simulink model "SM_Offshore_Windturbine"  (R2021a)
settings: Solver=ode4  StartTime=0.0  StopTime=par.sym.Ttot  FixedStep=par.sym.max_dt  MaxStep=par.sym.max_dt  RelTol=1e-3
model workspace: external: MATLAB File C:\Users\d053704\Desktop\MOST\Structure\CAD\CAD_DataFile.m (data not in the file)
undefined symbols (not defined in the file): par, smiData, X, Y, Z
libraries: sm_lib x50, simulink_extras x29, vrlib x18, nesl_utility x10, dspstat3 x9, sharedutil x5, eeGeneralControl x2
(part 4 of 4)

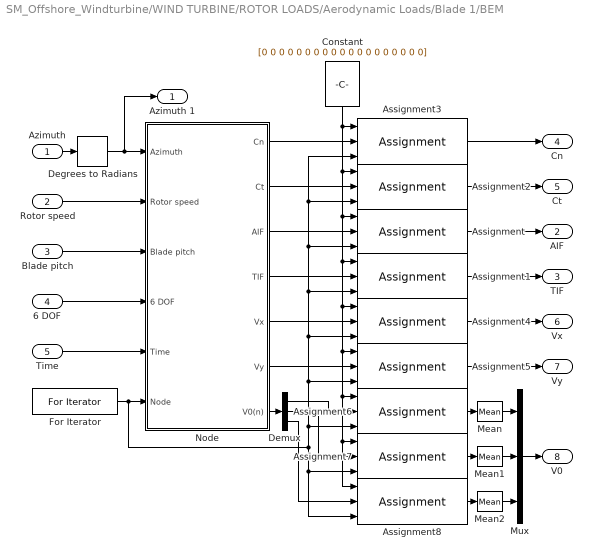
== system SM_Offshore_Windturbine/WIND TURBINE/ROTOR LOADS/Aerodynamic Loads/Blade 1/BEM ==
  Azimuth : Inport
  Rotor speed : Inport  Port=2
  Blade pitch : Inport  Port=3
  6 DOF : Inport  Port=4
  Time : Inport  Port=5
  Assignment{,1..8} (9 alike) : Assignment  IndexOptions=Index vector (port)  Indices=1  OutputSizes=1
  Constant : Constant  Value=[0 0 0 0 0 0 0 0 0 0 0 0 0 0 0 0 0 0 0]
  Degrees to Radians : simulink_extras/Transformations/Degrees to Radians
  Demux : Demux  Outputs=3
  For Iterator : ForIterator  IterationLimit=19  IterationVariableDataType=double
  Mean : dspstat3/Mean  run=off  InputProcessing=Columns as channels (frame based)  reset_popup=None  directionMode=Each column  dimension=1  roiEnable=off  roiType=Rectangles  roiPortion=Entire ROI  roiOutput=Individual statistics for each ROI  roiFlag=off  roundingMode=Floor  overflowMode=off  outputDataTypeStr=Inherit: Same as accumulator  outputMin=[]  outputMax=[]  outputLastDataTypeStr=Inherit: Same as accumulator
  Mean1 : dspstat3/Mean  run=off  InputProcessing=Columns as channels (frame based)  reset_popup=None  directionMode=Each column  dimension=1  roiEnable=off  roiType=Rectangles  roiPortion=Entire ROI  roiOutput=Individual statistics for each ROI  roiFlag=off  roundingMode=Floor  overflowMode=off  outputDataTypeStr=Inherit: Same as accumulator  outputMin=[]  outputMax=[]  outputLastDataTypeStr=Inherit: Same as accumulator
  Mean2 : dspstat3/Mean  run=off  InputProcessing=Columns as channels (frame based)  reset_popup=None  directionMode=Each column  dimension=1  roiEnable=off  roiType=Rectangles  roiPortion=Entire ROI  roiOutput=Individual statistics for each ROI  roiFlag=off  roundingMode=Floor  overflowMode=off  outputDataTypeStr=Inherit: Same as accumulator  outputMin=[]  outputMax=[]  outputLastDataTypeStr=Inherit: Same as accumulator
  Mux : Mux  Inputs=3
  Node : Subsystem
  Azimuth 1 : Outport  VectorParamsAs1DForOutWhenUnconnected=off
  AIF : Outport  Port=2  VectorParamsAs1DForOutWhenUnconnected=off
  TIF : Outport  Port=3  VectorParamsAs1DForOutWhenUnconnected=off
  Cn : Outport  Port=4  VectorParamsAs1DForOutWhenUnconnected=off
  Ct : Outport  Port=5  VectorParamsAs1DForOutWhenUnconnected=off
  Vx : Outport  Port=6  VectorParamsAs1DForOutWhenUnconnected=off
  Vy : Outport  Port=7  VectorParamsAs1DForOutWhenUnconnected=off
  V0 : Outport  Port=8  VectorParamsAs1DForOutWhenUnconnected=off
  wires:
  Blade pitch/1 -> Node/3(Blade pitch)
  6 DOF/1 -> Node/4(6 DOF)
  Time/1 -> Node/5(Time)
  Rotor speed/1 -> Node/2(Rotor speed)
  For Iterator/1 -> Node/6(Node), Assignment8/3, Assignment7/3, Assignment6/3, Assignment5/3, Assignment1/3, Assignment/3, Assignment3/3, Assignment2/3, Assignment4/3
  Assignment/1 -> AIF/1
  Assignment1/1 -> TIF/1
  Node/3(AIF) -> Assignment/2
  Node/4(TIF) -> Assignment1/2
  Node/2(Ct) -> Assignment2/2
  Node/1(Cn) -> Assignment3/2
  Node/5(Vx) -> Assignment4/2
  Node/6(Vy) -> Assignment5/2
  Constant/1 -> Assignment7/1, Assignment8/1, Assignment6/1, Assignment5/1, Assignment4/1, Assignment1/1, Assignment/1, Assignment2/1, Assignment3/1
  Assignment3/1 -> Cn/1
  Assignment2/1 -> Ct/1
  Assignment4/1 -> Vx/1
  Assignment5/1 -> Vy/1
  Node/7(V0(n)) -> Demux/1
  Demux/1 -> Assignment6/2
  Demux/3 -> Assignment8/2
  Demux/2 -> Assignment7/2
  Mux/1 -> V0/1
  Assignment6/1 -> Mean/1
  Assignment7/1 -> Mean1/1
  Assignment8/1 -> Mean2/1
  Mean/1 -> Mux/1
  Mean1/1 -> Mux/2
  Mean2/1 -> Mux/3
  Azimuth/1 -> Degrees to Radians/1
  Degrees to Radians/1 -> Node/1(Azimuth), Azimuth 1/1

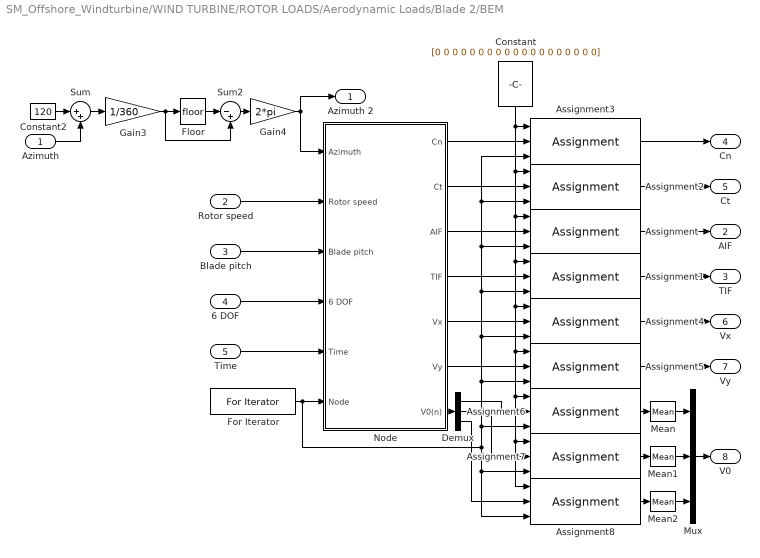
== system SM_Offshore_Windturbine/WIND TURBINE/ROTOR LOADS/Aerodynamic Loads/Blade 2/BEM ==
  Azimuth : Inport
  Rotor speed : Inport  Port=2
  Blade pitch : Inport  Port=3
  6 DOF : Inport  Port=4
  Time : Inport  Port=5
  Assignment{,1..8} (9 alike) : Assignment  IndexOptions=Index vector (port)  Indices=1  OutputSizes=1
  Constant : Constant  Value=[0 0 0 0 0 0 0 0 0 0 0 0 0 0 0 0 0 0 0]
  Constant2 : Constant  Value=120
  Demux : Demux  Outputs=3
  Floor : Rounding
  For Iterator : ForIterator  IterationLimit=19  IterationVariableDataType=double
  Gain3 : Gain  Gain=1/360
  Gain4 : Gain  Gain=2*pi
  Mean : dspstat3/Mean  run=off  InputProcessing=Columns as channels (frame based)  reset_popup=None  directionMode=Each column  dimension=1  roiEnable=off  roiType=Rectangles  roiPortion=Entire ROI  roiOutput=Individual statistics for each ROI  roiFlag=off  roundingMode=Floor  overflowMode=off  outputDataTypeStr=Inherit: Same as accumulator  outputMin=[]  outputMax=[]  outputLastDataTypeStr=Inherit: Same as accumulator
  Mean1 : dspstat3/Mean  run=off  InputProcessing=Columns as channels (frame based)  reset_popup=None  directionMode=Each column  dimension=1  roiEnable=off  roiType=Rectangles  roiPortion=Entire ROI  roiOutput=Individual statistics for each ROI  roiFlag=off  roundingMode=Floor  overflowMode=off  outputDataTypeStr=Inherit: Same as accumulator  outputMin=[]  outputMax=[]  outputLastDataTypeStr=Inherit: Same as accumulator
  Mean2 : dspstat3/Mean  run=off  InputProcessing=Columns as channels (frame based)  reset_popup=None  directionMode=Each column  dimension=1  roiEnable=off  roiType=Rectangles  roiPortion=Entire ROI  roiOutput=Individual statistics for each ROI  roiFlag=off  roundingMode=Floor  overflowMode=off  outputDataTypeStr=Inherit: Same as accumulator  outputMin=[]  outputMax=[]  outputLastDataTypeStr=Inherit: Same as accumulator
  Mux : Mux  Inputs=3
  Node : Subsystem
  Sum : Sum  Inputs=|++
  Sum2 : Sum  Inputs=|-+
  Azimuth 2 : Outport  VectorParamsAs1DForOutWhenUnconnected=off
  AIF : Outport  Port=2  VectorParamsAs1DForOutWhenUnconnected=off
  TIF : Outport  Port=3  VectorParamsAs1DForOutWhenUnconnected=off
  Cn : Outport  Port=4  VectorParamsAs1DForOutWhenUnconnected=off
  Ct : Outport  Port=5  VectorParamsAs1DForOutWhenUnconnected=off
  Vx : Outport  Port=6  VectorParamsAs1DForOutWhenUnconnected=off
  Vy : Outport  Port=7  VectorParamsAs1DForOutWhenUnconnected=off
  V0 : Outport  Port=8  VectorParamsAs1DForOutWhenUnconnected=off
  wires:
  Blade pitch/1 -> Node/3(Blade pitch)
  6 DOF/1 -> Node/4(6 DOF)
  Time/1 -> Node/5(Time)
  Rotor speed/1 -> Node/2(Rotor speed)
  Sum/1 -> Gain3/1
  Floor/1 -> Sum2/1
  Constant2/1 -> Sum/1
  Gain3/1 -> Sum2/2, Floor/1
  Sum2/1 -> Gain4/1
  Gain4/1 -> Node/1(Azimuth), Azimuth 2/1
  Azimuth/1 -> Sum/2
  Mean/1 -> Mux/1
  Node/7(V0(n)) -> Demux/1
  Node/5(Vx) -> Assignment4/2
  Mux/1 -> V0/1
  Assignment5/1 -> Vy/1
  Assignment4/1 -> Vx/1
  Constant/1 -> Assignment7/1, Assignment8/1, Assignment6/1, Assignment5/1, Assignment4/1, Assignment1/1, Assignment/1, Assignment2/1, Assignment3/1
  Demux/2 -> Assignment7/2
  Mean2/1 -> Mux/3
  Assignment8/1 -> Mean2/1
  Assignment6/1 -> Mean/1
  Assignment/1 -> AIF/1
  Node/4(TIF) -> Assignment1/2
  Assignment1/1 -> TIF/1
  Node/3(AIF) -> Assignment/2
  Demux/1 -> Assignment6/2
  Demux/3 -> Assignment8/2
  For Iterator/1 -> Node/6(Node), Assignment8/3, Assignment7/3, Assignment6/3, Assignment5/3, Assignment1/3, Assignment/3, Assignment3/3, Assignment2/3, Assignment4/3
  Node/2(Ct) -> Assignment2/2
  Node/1(Cn) -> Assignment3/2
  Assignment2/1 -> Ct/1
  Assignment3/1 -> Cn/1
  Node/6(Vy) -> Assignment5/2
  Mean1/1 -> Mux/2
  Assignment7/1 -> Mean1/1

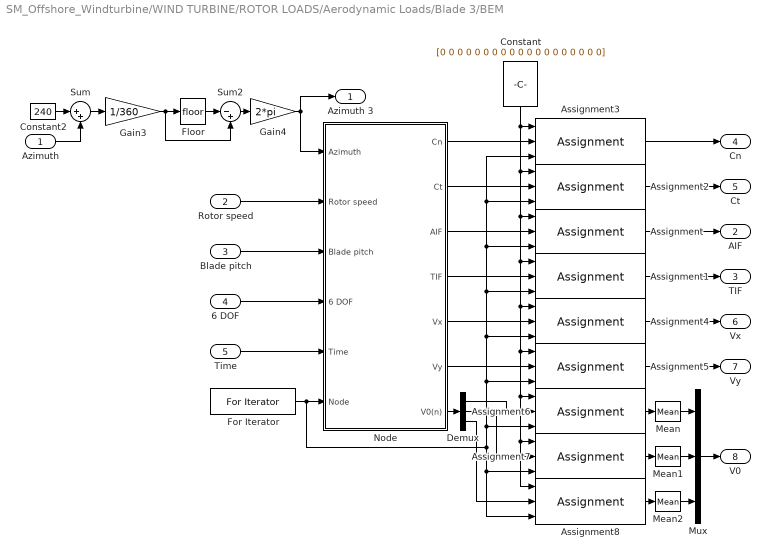
== system SM_Offshore_Windturbine/WIND TURBINE/ROTOR LOADS/Aerodynamic Loads/Blade 3/BEM ==
  Azimuth : Inport
  Rotor speed : Inport  Port=2
  Blade pitch : Inport  Port=3
  6 DOF : Inport  Port=4
  Time : Inport  Port=5
  Assignment{,1..8} (9 alike) : Assignment  IndexOptions=Index vector (port)  Indices=1  OutputSizes=1
  Constant : Constant  Value=[0 0 0 0 0 0 0 0 0 0 0 0 0 0 0 0 0 0 0]
  Constant2 : Constant  Value=240
  Demux : Demux  Outputs=3
  Floor : Rounding
  For Iterator : ForIterator  IterationLimit=19  IterationVariableDataType=double
  Gain3 : Gain  Gain=1/360
  Gain4 : Gain  Gain=2*pi
  Mean : dspstat3/Mean  run=off  InputProcessing=Columns as channels (frame based)  reset_popup=None  directionMode=Each column  dimension=1  roiEnable=off  roiType=Rectangles  roiPortion=Entire ROI  roiOutput=Individual statistics for each ROI  roiFlag=off  roundingMode=Floor  overflowMode=off  outputDataTypeStr=Inherit: Same as accumulator  outputMin=[]  outputMax=[]  outputLastDataTypeStr=Inherit: Same as accumulator
  Mean1 : dspstat3/Mean  run=off  InputProcessing=Columns as channels (frame based)  reset_popup=None  directionMode=Each column  dimension=1  roiEnable=off  roiType=Rectangles  roiPortion=Entire ROI  roiOutput=Individual statistics for each ROI  roiFlag=off  roundingMode=Floor  overflowMode=off  outputDataTypeStr=Inherit: Same as accumulator  outputMin=[]  outputMax=[]  outputLastDataTypeStr=Inherit: Same as accumulator
  Mean2 : dspstat3/Mean  run=off  InputProcessing=Columns as channels (frame based)  reset_popup=None  directionMode=Each column  dimension=1  roiEnable=off  roiType=Rectangles  roiPortion=Entire ROI  roiOutput=Individual statistics for each ROI  roiFlag=off  roundingMode=Floor  overflowMode=off  outputDataTypeStr=Inherit: Same as accumulator  outputMin=[]  outputMax=[]  outputLastDataTypeStr=Inherit: Same as accumulator
  Mux : Mux  Inputs=3
  Node : Subsystem
  Sum : Sum  Inputs=|++
  Sum2 : Sum  Inputs=|-+
  Azimuth 3 : Outport  VectorParamsAs1DForOutWhenUnconnected=off
  AIF : Outport  Port=2  VectorParamsAs1DForOutWhenUnconnected=off
  TIF : Outport  Port=3  VectorParamsAs1DForOutWhenUnconnected=off
  Cn : Outport  Port=4  VectorParamsAs1DForOutWhenUnconnected=off
  Ct : Outport  Port=5  VectorParamsAs1DForOutWhenUnconnected=off
  Vx : Outport  Port=6  VectorParamsAs1DForOutWhenUnconnected=off
  Vy : Outport  Port=7  VectorParamsAs1DForOutWhenUnconnected=off
  V0 : Outport  Port=8  VectorParamsAs1DForOutWhenUnconnected=off
  wires:
  Azimuth/1 -> Sum/2
  Gain4/1 -> Node/1(Azimuth), Azimuth 3/1
  Sum2/1 -> Gain4/1
  Gain3/1 -> Floor/1, Sum2/2
  Constant2/1 -> Sum/1
  Floor/1 -> Sum2/1
  Sum/1 -> Gain3/1
  Rotor speed/1 -> Node/2(Rotor speed)
  Time/1 -> Node/5(Time)
  6 DOF/1 -> Node/4(6 DOF)
  Blade pitch/1 -> Node/3(Blade pitch)
  Mean/1 -> Mux/1
  Node/7(V0(n)) -> Demux/1
  Node/5(Vx) -> Assignment4/2
  Mux/1 -> V0/1
  Assignment5/1 -> Vy/1
  Assignment4/1 -> Vx/1
  Constant/1 -> Assignment7/1, Assignment8/1, Assignment6/1, Assignment5/1, Assignment4/1, Assignment1/1, Assignment/1, Assignment2/1, Assignment3/1
  Demux/2 -> Assignment7/2
  Mean2/1 -> Mux/3
  Assignment8/1 -> Mean2/1
  Assignment6/1 -> Mean/1
  Assignment/1 -> AIF/1
  Node/4(TIF) -> Assignment1/2
  Assignment1/1 -> TIF/1
  Node/3(AIF) -> Assignment/2
  Demux/1 -> Assignment6/2
  Demux/3 -> Assignment8/2
  For Iterator/1 -> Node/6(Node), Assignment8/3, Assignment7/3, Assignment6/3, Assignment5/3, Assignment1/3, Assignment/3, Assignment3/3, Assignment2/3, Assignment4/3
  Node/2(Ct) -> Assignment2/2
  Node/1(Cn) -> Assignment3/2
  Assignment2/1 -> Ct/1
  Assignment3/1 -> Cn/1
  Node/6(Vy) -> Assignment5/2
  Mean1/1 -> Mux/2
  Assignment7/1 -> Mean1/1

== system SM_Offshore_Windturbine/WIND TURBINE/ROTOR LOADS/TowerBaseLoads/3D rotation matrix/If Action Subsystem ==
  Action Port : ActionPort  ActionPortLabel=if(u1 == 0)
  Constant : Constant  Value=[1 0 0; 0 1 0; 0 0 1]
  R : Outport  VectorParamsAs1DForOutWhenUnconnected=off
  wires:
  Constant/1 -> R/1

== system SM_Offshore_Windturbine/WIND TURBINE/ROTOR LOADS/TowerBaseLoads/3D rotation matrix/If Action Subsystem1 ==
  TETA : Inport
  rad : Inport  Port=2
  T : Inport  Port=3
  Action Port : ActionPort  ActionPortLabel=else
  Divide : Product  Inputs=//*
  R : Outport  VectorParamsAs1DForOutWhenUnconnected=off
  wires:
  T/1 -> Divide/3
  TETA/1 -> Divide/1
  rad/1 -> Divide/2
  Divide/1 -> R/1

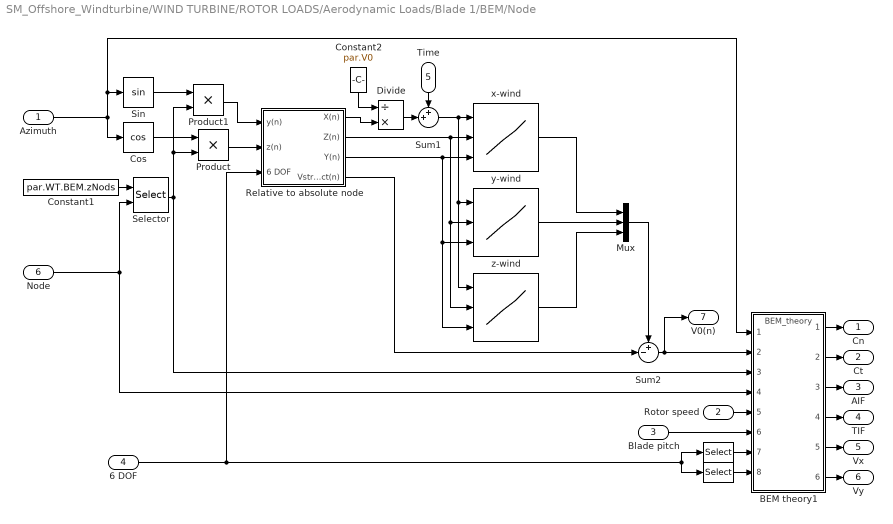
== system SM_Offshore_Windturbine/WIND TURBINE/ROTOR LOADS/Aerodynamic Loads/Blade 1/BEM/Node ==
  Azimuth : Inport
  Rotor speed : Inport  Port=2
  Blade pitch : Inport  Port=3
  6 DOF : Inport  Port=4
  Time : Inport  Port=5
  Node : Inport  Port=6
  " " : Selector  InputPortWidth=18  IndexOptions=Index vector (dialog)  Indices=6  OutputSizes=1
  "  " : Selector  InputPortWidth=18  IndexOptions=Index vector (dialog)  Indices=5  OutputSizes=1
  BEM theory1 : ModelReference  ModelNameDialog=BEM_theory.slxp  ModelReferenceVersion=5.17  CopyOfModelProtected=on
  Constant1 : Constant  Value=par.WT.BEM.zNods
  Constant2 : Constant  Value=par.V0  VectorParams1D=off
  Cos : Trigonometry  Operator=cos
  Divide : Product  Inputs=/*
  Mux : Mux  Inputs=3
  Product : Product
  Product1 : Product
  Relative to absolute node : Subsystem
  Selector : Selector  InputPortWidth=19  IndexOptions=Index vector (port)  Indices=Node  OutputSizes=1
  Sin : Trigonometry
  Sum1 : Sum  Inputs=++|
  Sum2 : Sum  Inputs=+-|
  x-wind : Lookup_n-D  NumberOfTableDimensions=3  BreakpointsForDimension1=par.wind.Time  BreakpointsForDimension2=par.wind.Zdiscr  BreakpointsForDimension3=par.wind.Ydiscr  BreakpointsForDimension4=par.WT.BEM.WINDANGLE  BreakpointsForDimension5=par.WT.BEM.AZIMUTH  BreakpointsForDimension6=par.WT.BEM.YAW  Table=par.wind.SpatialDiscrU  DiagnosticForOutOfRangeInput=Warning  RndMeth=Simplest  InputSameDT=on
      settings: InputPortMap=u0,u1,u2
  y-wind : Lookup_n-D  NumberOfTableDimensions=3  BreakpointsForDimension1=par.wind.Time  BreakpointsForDimension2=par.wind.Zdiscr  BreakpointsForDimension3=par.wind.Ydiscr  BreakpointsForDimension4=par.WT.BEM.WINDANGLE  BreakpointsForDimension5=par.WT.BEM.AZIMUTH  BreakpointsForDimension6=par.WT.BEM.YAW  Table=par.wind.SpatialDiscrV  DiagnosticForOutOfRangeInput=Warning  RndMeth=Simplest  InputSameDT=on
      settings: InputPortMap=u0,u1,u2
  z-wind : Lookup_n-D  NumberOfTableDimensions=3  BreakpointsForDimension1=par.wind.Time  BreakpointsForDimension2=par.wind.Zdiscr  BreakpointsForDimension3=par.wind.Ydiscr  BreakpointsForDimension4=par.WT.BEM.WINDANGLE  BreakpointsForDimension5=par.WT.BEM.AZIMUTH  BreakpointsForDimension6=par.WT.BEM.YAW  Table=par.wind.SpatialDiscrW  DiagnosticForOutOfRangeInput=Warning  RndMeth=Simplest  InputSameDT=on
      settings: InputPortMap=u0,u1,u2
  Cn : Outport  VectorParamsAs1DForOutWhenUnconnected=off
  Ct : Outport  Port=2  VectorParamsAs1DForOutWhenUnconnected=off
  AIF : Outport  Port=3  VectorParamsAs1DForOutWhenUnconnected=off
  TIF : Outport  Port=4  VectorParamsAs1DForOutWhenUnconnected=off
  Vx : Outport  Port=5  VectorParamsAs1DForOutWhenUnconnected=off
  Vy : Outport  Port=6  VectorParamsAs1DForOutWhenUnconnected=off
  V0(n) : Outport  Port=7  VectorParamsAs1DForOutWhenUnconnected=off
  wires:
  BEM theory1/2 -> Ct/1
  BEM theory1/1 -> Cn/1
  Divide/1 -> Sum1/2
  Product/1 -> Relative to absolute node/2(z(n))
  Cos/1 -> Product/1
  x-wind/1 -> Mux/1
  Product1/1 -> Relative to absolute node/1(y(n))
  y-wind/1 -> Mux/2
  Relative to absolute node/1(X(n)) -> Divide/2
  Relative to absolute node/3(Y(n)) -> x-wind/3, z-wind/3, y-wind/3
  Sum1/1 -> z-wind/1, y-wind/1, x-wind/1
  Constant2/1 -> Divide/1
  Azimuth/1 -> BEM theory1/1, Sin/1, Cos/1
  Selector/1 -> BEM theory1/3, Product/2, Product1/2
  z-wind/1 -> Mux/3
  Sin/1 -> Product1/1
  "  "/1 -> BEM theory1/7
  " "/1 -> BEM theory1/8
  Rotor speed/1 -> BEM theory1/5
  6 DOF/1 -> Relative to absolute node/3(6 DOF), " "/1, "  "/1
  Blade pitch/1 -> BEM theory1/6
  Node/1 -> BEM theory1/4, Selector/2
  Constant1/1 -> Selector/1
  Time/1 -> Sum1/1
  BEM theory1/3 -> AIF/1
  Relative to absolute node/4(Vstruct(n)) -> Sum2/2
  BEM theory1/4 -> TIF/1
  BEM theory1/6 -> Vy/1
  BEM theory1/5 -> Vx/1
  Sum2/1 -> BEM theory1/2, V0(n)/1
  Relative to absolute node/2(Z(n)) -> z-wind/2, y-wind/2, x-wind/2
  Mux/1 -> Sum2/1

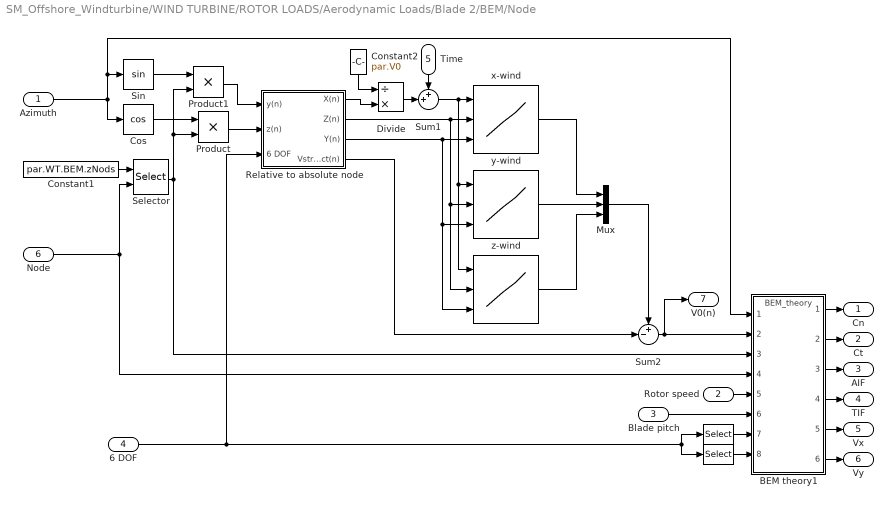
== system SM_Offshore_Windturbine/WIND TURBINE/ROTOR LOADS/Aerodynamic Loads/Blade 2/BEM/Node ==
  Azimuth : Inport
  Rotor speed : Inport  Port=2
  Blade pitch : Inport  Port=3
  6 DOF : Inport  Port=4
  Time : Inport  Port=5
  Node : Inport  Port=6
  " " : Selector  InputPortWidth=18  IndexOptions=Index vector (dialog)  Indices=6  OutputSizes=1
  "  " : Selector  InputPortWidth=18  IndexOptions=Index vector (dialog)  Indices=5  OutputSizes=1
  BEM theory1 : ModelReference  ModelNameDialog=BEM_theory.slxp  ModelReferenceVersion=5.17  CopyOfModelProtected=on
  Constant1 : Constant  Value=par.WT.BEM.zNods
  Constant2 : Constant  Value=par.V0  VectorParams1D=off
  Cos : Trigonometry  Operator=cos
  Divide : Product  Inputs=/*
  Mux : Mux  Inputs=3
  Product : Product
  Product1 : Product
  Relative to absolute node : Subsystem
  Selector : Selector  InputPortWidth=19  IndexOptions=Index vector (port)  Indices=Node  OutputSizes=1
  Sin : Trigonometry
  Sum1 : Sum  Inputs=++|
  Sum2 : Sum  Inputs=+-|
  x-wind : Lookup_n-D  NumberOfTableDimensions=3  BreakpointsForDimension1=par.wind.Time  BreakpointsForDimension2=par.wind.Zdiscr  BreakpointsForDimension3=par.wind.Ydiscr  BreakpointsForDimension4=par.WT.BEM.WINDANGLE  BreakpointsForDimension5=par.WT.BEM.AZIMUTH  BreakpointsForDimension6=par.WT.BEM.YAW  Table=par.wind.SpatialDiscrU  DiagnosticForOutOfRangeInput=Warning  RndMeth=Simplest  InputSameDT=on
      settings: InputPortMap=u0,u1,u2
  y-wind : Lookup_n-D  NumberOfTableDimensions=3  BreakpointsForDimension1=par.wind.Time  BreakpointsForDimension2=par.wind.Zdiscr  BreakpointsForDimension3=par.wind.Ydiscr  BreakpointsForDimension4=par.WT.BEM.WINDANGLE  BreakpointsForDimension5=par.WT.BEM.AZIMUTH  BreakpointsForDimension6=par.WT.BEM.YAW  Table=par.wind.SpatialDiscrV  DiagnosticForOutOfRangeInput=Warning  RndMeth=Simplest  InputSameDT=on
      settings: InputPortMap=u0,u1,u2
  z-wind : Lookup_n-D  NumberOfTableDimensions=3  BreakpointsForDimension1=par.wind.Time  BreakpointsForDimension2=par.wind.Zdiscr  BreakpointsForDimension3=par.wind.Ydiscr  BreakpointsForDimension4=par.WT.BEM.WINDANGLE  BreakpointsForDimension5=par.WT.BEM.AZIMUTH  BreakpointsForDimension6=par.WT.BEM.YAW  Table=par.wind.SpatialDiscrW  DiagnosticForOutOfRangeInput=Warning  RndMeth=Simplest  InputSameDT=on
      settings: InputPortMap=u0,u1,u2
  Cn : Outport  VectorParamsAs1DForOutWhenUnconnected=off
  Ct : Outport  Port=2  VectorParamsAs1DForOutWhenUnconnected=off
  AIF : Outport  Port=3  VectorParamsAs1DForOutWhenUnconnected=off
  TIF : Outport  Port=4  VectorParamsAs1DForOutWhenUnconnected=off
  Vx : Outport  Port=5  VectorParamsAs1DForOutWhenUnconnected=off
  Vy : Outport  Port=6  VectorParamsAs1DForOutWhenUnconnected=off
  V0(n) : Outport  Port=7  VectorParamsAs1DForOutWhenUnconnected=off
  wires:
  BEM theory1/2 -> Ct/1
  BEM theory1/1 -> Cn/1
  Divide/1 -> Sum1/2
  Product/1 -> Relative to absolute node/2(z(n))
  Cos/1 -> Product/1
  x-wind/1 -> Mux/1
  Product1/1 -> Relative to absolute node/1(y(n))
  y-wind/1 -> Mux/2
  Relative to absolute node/1(X(n)) -> Divide/2
  Relative to absolute node/3(Y(n)) -> x-wind/3, z-wind/3, y-wind/3
  Sum1/1 -> z-wind/1, y-wind/1, x-wind/1
  Constant2/1 -> Divide/1
  Azimuth/1 -> BEM theory1/1, Sin/1, Cos/1
  Selector/1 -> BEM theory1/3, Product/2, Product1/2
  z-wind/1 -> Mux/3
  Sin/1 -> Product1/1
  "  "/1 -> BEM theory1/7
  " "/1 -> BEM theory1/8
  Rotor speed/1 -> BEM theory1/5
  6 DOF/1 -> Relative to absolute node/3(6 DOF), " "/1, "  "/1
  Blade pitch/1 -> BEM theory1/6
  Node/1 -> BEM theory1/4, Selector/2
  Constant1/1 -> Selector/1
  Time/1 -> Sum1/1
  BEM theory1/3 -> AIF/1
  Relative to absolute node/4(Vstruct(n)) -> Sum2/2
  BEM theory1/4 -> TIF/1
  BEM theory1/6 -> Vy/1
  BEM theory1/5 -> Vx/1
  Sum2/1 -> BEM theory1/2, V0(n)/1
  Relative to absolute node/2(Z(n)) -> z-wind/2, y-wind/2, x-wind/2
  Mux/1 -> Sum2/1

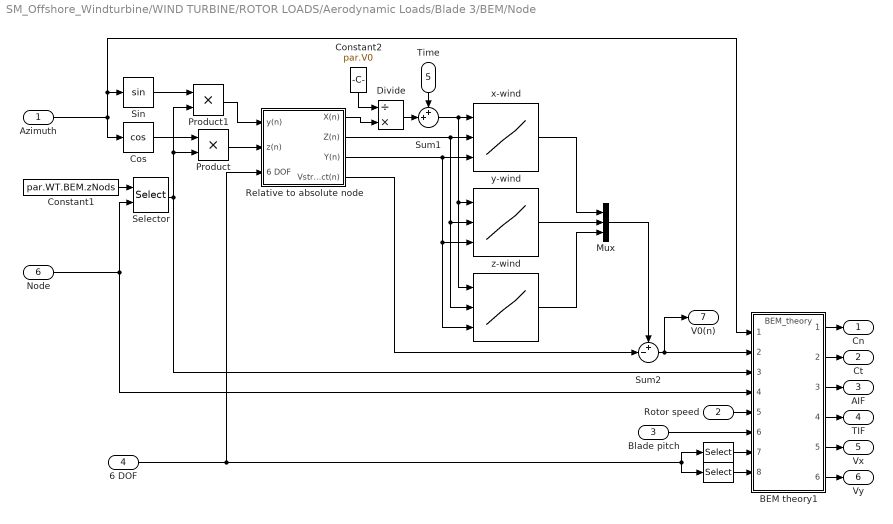
== system SM_Offshore_Windturbine/WIND TURBINE/ROTOR LOADS/Aerodynamic Loads/Blade 3/BEM/Node ==
  Azimuth : Inport
  Rotor speed : Inport  Port=2
  Blade pitch : Inport  Port=3
  6 DOF : Inport  Port=4
  Time : Inport  Port=5
  Node : Inport  Port=6
  " " : Selector  InputPortWidth=18  IndexOptions=Index vector (dialog)  Indices=6  OutputSizes=1
  "  " : Selector  InputPortWidth=18  IndexOptions=Index vector (dialog)  Indices=5  OutputSizes=1
  BEM theory1 : ModelReference  ModelNameDialog=BEM_theory.slxp  ModelReferenceVersion=5.17  CopyOfModelProtected=on
  Constant1 : Constant  Value=par.WT.BEM.zNods
  Constant2 : Constant  Value=par.V0  VectorParams1D=off
  Cos : Trigonometry  Operator=cos
  Divide : Product  Inputs=/*
  Mux : Mux  Inputs=3
  Product : Product
  Product1 : Product
  Relative to absolute node : Subsystem
  Selector : Selector  InputPortWidth=19  IndexOptions=Index vector (port)  Indices=Node  OutputSizes=1
  Sin : Trigonometry
  Sum1 : Sum  Inputs=++|
  Sum2 : Sum  Inputs=+-|
  x-wind : Lookup_n-D  NumberOfTableDimensions=3  BreakpointsForDimension1=par.wind.Time  BreakpointsForDimension2=par.wind.Zdiscr  BreakpointsForDimension3=par.wind.Ydiscr  BreakpointsForDimension4=par.WT.BEM.WINDANGLE  BreakpointsForDimension5=par.WT.BEM.AZIMUTH  BreakpointsForDimension6=par.WT.BEM.YAW  Table=par.wind.SpatialDiscrU  DiagnosticForOutOfRangeInput=Warning  RndMeth=Simplest  InputSameDT=on
      settings: InputPortMap=u0,u1,u2
  y-wind : Lookup_n-D  NumberOfTableDimensions=3  BreakpointsForDimension1=par.wind.Time  BreakpointsForDimension2=par.wind.Zdiscr  BreakpointsForDimension3=par.wind.Ydiscr  BreakpointsForDimension4=par.WT.BEM.WINDANGLE  BreakpointsForDimension5=par.WT.BEM.AZIMUTH  BreakpointsForDimension6=par.WT.BEM.YAW  Table=par.wind.SpatialDiscrV  DiagnosticForOutOfRangeInput=Warning  RndMeth=Simplest  InputSameDT=on
      settings: InputPortMap=u0,u1,u2
  z-wind : Lookup_n-D  NumberOfTableDimensions=3  BreakpointsForDimension1=par.wind.Time  BreakpointsForDimension2=par.wind.Zdiscr  BreakpointsForDimension3=par.wind.Ydiscr  BreakpointsForDimension4=par.WT.BEM.WINDANGLE  BreakpointsForDimension5=par.WT.BEM.AZIMUTH  BreakpointsForDimension6=par.WT.BEM.YAW  Table=par.wind.SpatialDiscrW  DiagnosticForOutOfRangeInput=Warning  RndMeth=Simplest  InputSameDT=on
      settings: InputPortMap=u0,u1,u2
  Cn : Outport  VectorParamsAs1DForOutWhenUnconnected=off
  Ct : Outport  Port=2  VectorParamsAs1DForOutWhenUnconnected=off
  AIF : Outport  Port=3  VectorParamsAs1DForOutWhenUnconnected=off
  TIF : Outport  Port=4  VectorParamsAs1DForOutWhenUnconnected=off
  Vx : Outport  Port=5  VectorParamsAs1DForOutWhenUnconnected=off
  Vy : Outport  Port=6  VectorParamsAs1DForOutWhenUnconnected=off
  V0(n) : Outport  Port=7  VectorParamsAs1DForOutWhenUnconnected=off
  wires:
  BEM theory1/2 -> Ct/1
  BEM theory1/1 -> Cn/1
  Divide/1 -> Sum1/2
  Product/1 -> Relative to absolute node/2(z(n))
  Cos/1 -> Product/1
  x-wind/1 -> Mux/1
  Product1/1 -> Relative to absolute node/1(y(n))
  y-wind/1 -> Mux/2
  Relative to absolute node/1(X(n)) -> Divide/2
  Relative to absolute node/3(Y(n)) -> x-wind/3, z-wind/3, y-wind/3
  Sum1/1 -> z-wind/1, y-wind/1, x-wind/1
  Constant2/1 -> Divide/1
  Azimuth/1 -> BEM theory1/1, Sin/1, Cos/1
  Selector/1 -> BEM theory1/3, Product/2, Product1/2
  z-wind/1 -> Mux/3
  Sin/1 -> Product1/1
  "  "/1 -> BEM theory1/7
  " "/1 -> BEM theory1/8
  Rotor speed/1 -> BEM theory1/5
  6 DOF/1 -> Relative to absolute node/3(6 DOF), " "/1, "  "/1
  Blade pitch/1 -> BEM theory1/6
  Node/1 -> BEM theory1/4, Selector/2
  Constant1/1 -> Selector/1
  Time/1 -> Sum1/1
  BEM theory1/3 -> AIF/1
  Relative to absolute node/4(Vstruct(n)) -> Sum2/2
  BEM theory1/4 -> TIF/1
  BEM theory1/6 -> Vy/1
  BEM theory1/5 -> Vx/1
  Sum2/1 -> BEM theory1/2, V0(n)/1
  Relative to absolute node/2(Z(n)) -> z-wind/2, y-wind/2, x-wind/2
  Mux/1 -> Sum2/1

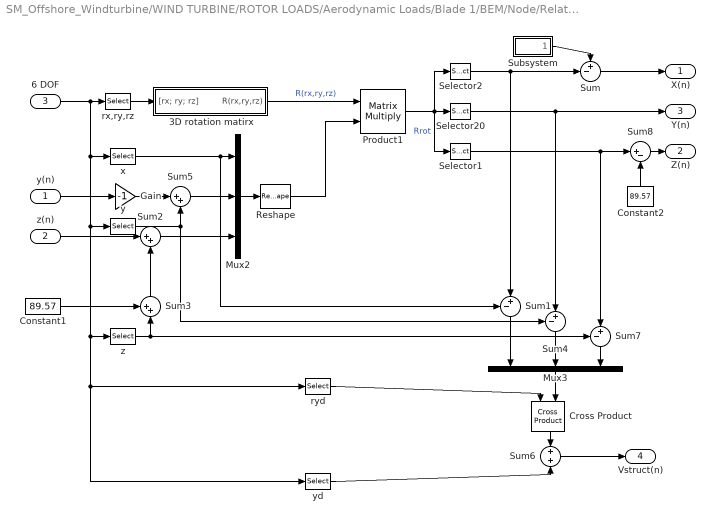
== system SM_Offshore_Windturbine/WIND TURBINE/ROTOR LOADS/Aerodynamic Loads/Blade 1/BEM/Node/Relative to absolute node ==
  y(n) : Inport
  z(n) : Inport  Port=2
  6 DOF : Inport  Port=3
  3D rotation matirx : Subsystem
  Constant1 : Constant  Value=89.57
  Constant2 : Constant  Value=89.57
  Cross Product : vrlib/Utilities/Cross Product
  Gain : Gain  Gain=-1
  Mux2 : Mux  Inputs=3
  Mux3 : Mux  Inputs=3
  Product1 : Product  Multiplication=Matrix(*)
  Reshape : Reshape
  Selector1 : Selector  InputPortWidth=3  IndexOptions=Index vector (dialog)  Indices=3  OutputSizes=1
  Selector2 : Selector  InputPortWidth=3  IndexOptions=Index vector (dialog)  Indices=1  OutputSizes=1
  Selector20 : Selector  InputPortWidth=3  IndexOptions=Index vector (dialog)  Indices=2  OutputSizes=1
  Subsystem : Subsystem
  Sum : Sum  Inputs=+-|
  Sum1 : Sum  Inputs=-+|
  Sum2 : Sum  Inputs=|++
  Sum3 : Sum  Inputs=++|
  Sum4 : Sum  Inputs=-+|
  Sum5 : Sum  Inputs=|++
  Sum6 : Sum
  Sum7 : Sum  Inputs=-+|
  Sum8 : Sum  Inputs=|+-
  "rx,ry,rz " : Selector  InputPortWidth=18  IndexOptions=Index vector (dialog)  Indices=[4 5 6]  OutputSizes=1
  ryd : Selector  InputPortWidth=18  IndexOptions=Index vector (dialog)  Indices=[10 11 12]  OutputSizes=1
  x : Selector  InputPortWidth=18  IndexOptions=Index vector (dialog)  Indices=1  OutputSizes=1
  y : Selector  InputPortWidth=18  IndexOptions=Index vector (dialog)  Indices=2  OutputSizes=1
  yd : Selector  InputPortWidth=18  IndexOptions=Index vector (dialog)  Indices=[7 8 9]  OutputSizes=1
  z : Selector  InputPortWidth=18  IndexOptions=Index vector (dialog)  Indices=3  OutputSizes=1
  X(n) : Outport  VectorParamsAs1DForOutWhenUnconnected=off
  Z(n) : Outport  Port=2  VectorParamsAs1DForOutWhenUnconnected=off
  Y(n) : Outport  Port=3  VectorParamsAs1DForOutWhenUnconnected=off
  Vstruct(n) : Outport  Port=4  VectorParamsAs1DForOutWhenUnconnected=off
  wires:
  Sum2/1 -> Mux2/3
  z(n)/1 -> Sum2/1
  z/1 -> Sum7/1, Sum3/2
  Reshape/1 -> Product1/2
  Mux2/1 -> Reshape/1
  6 DOF/1 -> yd/1, ryd/1, z/1, y/1, x/1, "rx,ry,rz "/1
  "rx,ry,rz "/1 -> 3D rotation matirx/1("[rx; ry; rz]")
  Product1/1 -> Selector20/1, Selector2/1, Selector1/1  "Rrot"
  Selector1/1 -> Sum8/1, Sum7/2
  Cross Product/1 -> Sum6/1
  yd/1 -> Sum6/2
  Sum6/1 -> Vstruct(n)/1
  ryd/1 -> Cross Product/1
  Mux3/1 -> Cross Product/2
  Selector2/1 -> Sum/2, Sum1/2
  Selector20/1 -> Sum4/2, Y(n)/1
  3D rotation matirx/1(R(rx,ry,rz)) -> Product1/1  "R(rx,ry,rz)"
  y(n)/1 -> Gain/1
  x/1 -> Sum1/1, Mux2/1
  Sum5/1 -> Mux2/2
  y/1 -> Sum4/1, Sum5/2
  Gain/1 -> Sum5/1
  Constant1/1 -> Sum3/1
  Sum3/1 -> Sum2/2
  Sum7/1 -> Mux3/3
  Sum4/1 -> Mux3/2
  Sum1/1 -> Mux3/1
  Sum/1 -> X(n)/1
  Sum8/1 -> Z(n)/1
  Constant2/1 -> Sum8/2
  Subsystem/1(X_iniz) -> Sum/1

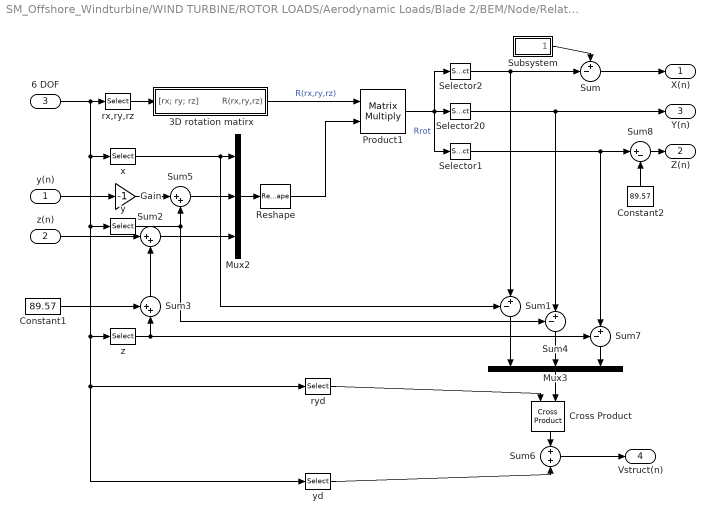
== system SM_Offshore_Windturbine/WIND TURBINE/ROTOR LOADS/Aerodynamic Loads/Blade 2/BEM/Node/Relative to absolute node ==
  y(n) : Inport
  z(n) : Inport  Port=2
  6 DOF : Inport  Port=3
  3D rotation matirx : Subsystem
  Constant1 : Constant  Value=89.57
  Constant2 : Constant  Value=89.57
  Cross Product : vrlib/Utilities/Cross Product
  Gain : Gain  Gain=-1
  Mux2 : Mux  Inputs=3
  Mux3 : Mux  Inputs=3
  Product1 : Product  Multiplication=Matrix(*)
  Reshape : Reshape
  Selector1 : Selector  InputPortWidth=3  IndexOptions=Index vector (dialog)  Indices=3  OutputSizes=1
  Selector2 : Selector  InputPortWidth=3  IndexOptions=Index vector (dialog)  Indices=1  OutputSizes=1
  Selector20 : Selector  InputPortWidth=3  IndexOptions=Index vector (dialog)  Indices=2  OutputSizes=1
  Subsystem : Subsystem
  Sum : Sum  Inputs=+-|
  Sum1 : Sum  Inputs=-+|
  Sum2 : Sum  Inputs=|++
  Sum3 : Sum  Inputs=++|
  Sum4 : Sum  Inputs=-+|
  Sum5 : Sum  Inputs=|++
  Sum6 : Sum
  Sum7 : Sum  Inputs=-+|
  Sum8 : Sum  Inputs=|+-
  "rx,ry,rz " : Selector  InputPortWidth=18  IndexOptions=Index vector (dialog)  Indices=[4 5 6]  OutputSizes=1
  ryd : Selector  InputPortWidth=18  IndexOptions=Index vector (dialog)  Indices=[10 11 12]  OutputSizes=1
  x : Selector  InputPortWidth=18  IndexOptions=Index vector (dialog)  Indices=1  OutputSizes=1
  y : Selector  InputPortWidth=18  IndexOptions=Index vector (dialog)  Indices=2  OutputSizes=1
  yd : Selector  InputPortWidth=18  IndexOptions=Index vector (dialog)  Indices=[7 8 9]  OutputSizes=1
  z : Selector  InputPortWidth=18  IndexOptions=Index vector (dialog)  Indices=3  OutputSizes=1
  X(n) : Outport  VectorParamsAs1DForOutWhenUnconnected=off
  Z(n) : Outport  Port=2  VectorParamsAs1DForOutWhenUnconnected=off
  Y(n) : Outport  Port=3  VectorParamsAs1DForOutWhenUnconnected=off
  Vstruct(n) : Outport  Port=4  VectorParamsAs1DForOutWhenUnconnected=off
  wires:
  Sum2/1 -> Mux2/3
  z(n)/1 -> Sum2/1
  z/1 -> Sum7/1, Sum3/2
  Reshape/1 -> Product1/2
  Mux2/1 -> Reshape/1
  6 DOF/1 -> yd/1, ryd/1, z/1, y/1, x/1, "rx,ry,rz "/1
  "rx,ry,rz "/1 -> 3D rotation matirx/1("[rx; ry; rz]")
  Product1/1 -> Selector20/1, Selector2/1, Selector1/1  "Rrot"
  Selector1/1 -> Sum8/1, Sum7/2
  Cross Product/1 -> Sum6/1
  yd/1 -> Sum6/2
  Sum6/1 -> Vstruct(n)/1
  ryd/1 -> Cross Product/1
  Mux3/1 -> Cross Product/2
  Selector2/1 -> Sum/2, Sum1/2
  Selector20/1 -> Sum4/2, Y(n)/1
  3D rotation matirx/1(R(rx,ry,rz)) -> Product1/1  "R(rx,ry,rz)"
  y(n)/1 -> Gain/1
  x/1 -> Sum1/1, Mux2/1
  Sum5/1 -> Mux2/2
  y/1 -> Sum4/1, Sum5/2
  Gain/1 -> Sum5/1
  Constant1/1 -> Sum3/1
  Sum3/1 -> Sum2/2
  Sum7/1 -> Mux3/3
  Sum4/1 -> Mux3/2
  Sum1/1 -> Mux3/1
  Sum/1 -> X(n)/1
  Sum8/1 -> Z(n)/1
  Constant2/1 -> Sum8/2
  Subsystem/1(X_iniz) -> Sum/1

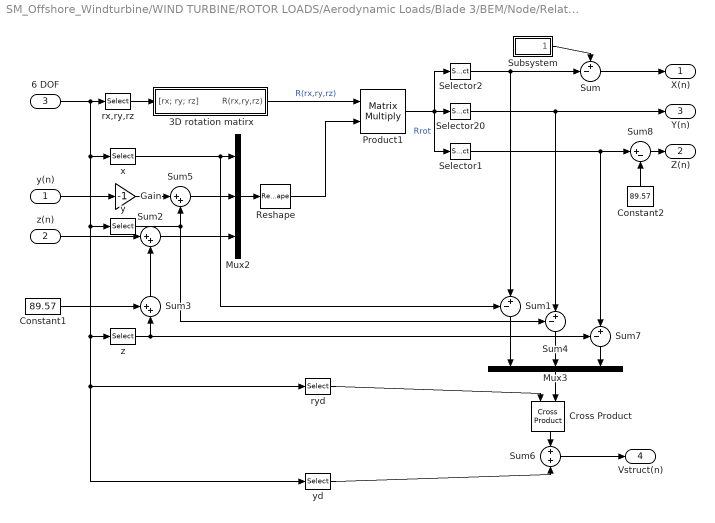
== system SM_Offshore_Windturbine/WIND TURBINE/ROTOR LOADS/Aerodynamic Loads/Blade 3/BEM/Node/Relative to absolute node ==
  y(n) : Inport
  z(n) : Inport  Port=2
  6 DOF : Inport  Port=3
  3D rotation matirx : Subsystem
  Constant1 : Constant  Value=89.57
  Constant2 : Constant  Value=89.57
  Cross Product : vrlib/Utilities/Cross Product
  Gain : Gain  Gain=-1
  Mux2 : Mux  Inputs=3
  Mux3 : Mux  Inputs=3
  Product1 : Product  Multiplication=Matrix(*)
  Reshape : Reshape
  Selector1 : Selector  InputPortWidth=3  IndexOptions=Index vector (dialog)  Indices=3  OutputSizes=1
  Selector2 : Selector  InputPortWidth=3  IndexOptions=Index vector (dialog)  Indices=1  OutputSizes=1
  Selector20 : Selector  InputPortWidth=3  IndexOptions=Index vector (dialog)  Indices=2  OutputSizes=1
  Subsystem : Subsystem
  Sum : Sum  Inputs=+-|
  Sum1 : Sum  Inputs=-+|
  Sum2 : Sum  Inputs=|++
  Sum3 : Sum  Inputs=++|
  Sum4 : Sum  Inputs=-+|
  Sum5 : Sum  Inputs=|++
  Sum6 : Sum
  Sum7 : Sum  Inputs=-+|
  Sum8 : Sum  Inputs=|+-
  "rx,ry,rz " : Selector  InputPortWidth=18  IndexOptions=Index vector (dialog)  Indices=[4 5 6]  OutputSizes=1
  ryd : Selector  InputPortWidth=18  IndexOptions=Index vector (dialog)  Indices=[10 11 12]  OutputSizes=1
  x : Selector  InputPortWidth=18  IndexOptions=Index vector (dialog)  Indices=1  OutputSizes=1
  y : Selector  InputPortWidth=18  IndexOptions=Index vector (dialog)  Indices=2  OutputSizes=1
  yd : Selector  InputPortWidth=18  IndexOptions=Index vector (dialog)  Indices=[7 8 9]  OutputSizes=1
  z : Selector  InputPortWidth=18  IndexOptions=Index vector (dialog)  Indices=3  OutputSizes=1
  X(n) : Outport  VectorParamsAs1DForOutWhenUnconnected=off
  Z(n) : Outport  Port=2  VectorParamsAs1DForOutWhenUnconnected=off
  Y(n) : Outport  Port=3  VectorParamsAs1DForOutWhenUnconnected=off
  Vstruct(n) : Outport  Port=4  VectorParamsAs1DForOutWhenUnconnected=off
  wires:
  Sum2/1 -> Mux2/3
  z(n)/1 -> Sum2/1
  z/1 -> Sum7/1, Sum3/2
  Reshape/1 -> Product1/2
  Mux2/1 -> Reshape/1
  6 DOF/1 -> yd/1, ryd/1, z/1, y/1, x/1, "rx,ry,rz "/1
  "rx,ry,rz "/1 -> 3D rotation matirx/1("[rx; ry; rz]")
  Product1/1 -> Selector20/1, Selector2/1, Selector1/1  "Rrot"
  Selector1/1 -> Sum8/1, Sum7/2
  Cross Product/1 -> Sum6/1
  yd/1 -> Sum6/2
  Sum6/1 -> Vstruct(n)/1
  ryd/1 -> Cross Product/1
  Mux3/1 -> Cross Product/2
  Selector2/1 -> Sum/2, Sum1/2
  Selector20/1 -> Sum4/2, Y(n)/1
  3D rotation matirx/1(R(rx,ry,rz)) -> Product1/1  "R(rx,ry,rz)"
  y(n)/1 -> Gain/1
  x/1 -> Sum1/1, Mux2/1
  Sum5/1 -> Mux2/2
  y/1 -> Sum4/1, Sum5/2
  Gain/1 -> Sum5/1
  Constant1/1 -> Sum3/1
  Sum3/1 -> Sum2/2
  Sum7/1 -> Mux3/3
  Sum4/1 -> Mux3/2
  Sum1/1 -> Mux3/1
  Sum/1 -> X(n)/1
  Sum8/1 -> Z(n)/1
  Constant2/1 -> Sum8/2
  Subsystem/1(X_iniz) -> Sum/1

== system SM_Offshore_Windturbine/WIND TURBINE/ROTOR LOADS/Aerodynamic Loads/Blade 1/BEM/Node/Relative to absolute node/3D rotation matirx ==
  "[rx; ry; rz]" : Inport  PortDimensions=3
  Create 3x3 Matrix : sharedutil/Create 3x3 Matrix  aMode=aMode
      settings: SourceProductBaseCode=AE,PW,DR,MT,UV,VE
  Fcn11 : Fcn  Expr=u(5)*u(6)
  Fcn12 : Fcn  Expr=u(6)*u(1)*u(2) - u(4)*u(3)
  Fcn13 : Fcn  Expr=u(4)*u(6)*u(2) + u(1)*u(3)
  Fcn21 : Fcn  Expr=u(5)*u(3)
  Fcn22 : Fcn  Expr=u(4)*u(6) + u(1)*u(2) *u(3)
  Fcn23 : Fcn  Expr=-u(6)*u(1) + u(4)*u(2) *u(3)
  Fcn31 : Fcn  Expr=-u(2)
  Fcn32 : Fcn  Expr=u(5)*u(1)
  Fcn33 : Fcn  Expr=u(4)*u(5)
  Mux : Mux  Inputs=2
  sincos : Trigonometry  Operator=sincos
  R(rx,ry,rz) : Outport  PortDimensions=[3,3]  VectorParamsAs1DForOutWhenUnconnected=off
  wires:
  "[rx; ry; rz]"/1 -> sincos/1
  Create 3x3 Matrix/1 -> R(rx,ry,rz)/1
  sincos/1 -> Mux/1
  sincos/2 -> Mux/2
  Mux/1 -> Fcn11/1, Fcn12/1, Fcn13/1, Fcn21/1, Fcn32/1, Fcn33/1, Fcn31/1, Fcn23/1, Fcn22/1
  Fcn11/1 -> Create 3x3 Matrix/1
  Fcn12/1 -> Create 3x3 Matrix/2
  Fcn13/1 -> Create 3x3 Matrix/3
  Fcn31/1 -> Create 3x3 Matrix/7
  Fcn22/1 -> Create 3x3 Matrix/5
  Fcn32/1 -> Create 3x3 Matrix/8
  Fcn33/1 -> Create 3x3 Matrix/9
  Fcn21/1 -> Create 3x3 Matrix/4
  Fcn23/1 -> Create 3x3 Matrix/6

== system SM_Offshore_Windturbine/WIND TURBINE/ROTOR LOADS/Aerodynamic Loads/Blade 1/BEM/Node/Relative to absolute node/Subsystem ==
  Constant6 : Constant  Value=12
  Constant8 : Constant  Value=12.083
  Constant9 : Constant  Value=0.5
  Product3 : Product  Inputs=3
  X_iniz : Outport
  wires:
  Product3/1 -> X_iniz/1
  Constant8/1 -> Product3/2
  Constant6/1 -> Product3/3
  Constant9/1 -> Product3/1

== system SM_Offshore_Windturbine/WIND TURBINE/ROTOR LOADS/Aerodynamic Loads/Blade 2/BEM/Node/Relative to absolute node/3D rotation matirx ==
  "[rx; ry; rz]" : Inport  PortDimensions=3
  Create 3x3 Matrix : sharedutil/Create 3x3 Matrix  aMode=aMode
      settings: SourceProductBaseCode=AE,PW,DR,MT,UV,VE
  Fcn11 : Fcn  Expr=u(5)*u(6)
  Fcn12 : Fcn  Expr=u(6)*u(1)*u(2) - u(4)*u(3)
  Fcn13 : Fcn  Expr=u(4)*u(6)*u(2) + u(1)*u(3)
  Fcn21 : Fcn  Expr=u(5)*u(3)
  Fcn22 : Fcn  Expr=u(4)*u(6) + u(1)*u(2) *u(3)
  Fcn23 : Fcn  Expr=-u(6)*u(1) + u(4)*u(2) *u(3)
  Fcn31 : Fcn  Expr=-u(2)
  Fcn32 : Fcn  Expr=u(5)*u(1)
  Fcn33 : Fcn  Expr=u(4)*u(5)
  Mux : Mux  Inputs=2
  sincos : Trigonometry  Operator=sincos
  R(rx,ry,rz) : Outport  PortDimensions=[3,3]  VectorParamsAs1DForOutWhenUnconnected=off
  wires:
  "[rx; ry; rz]"/1 -> sincos/1
  Create 3x3 Matrix/1 -> R(rx,ry,rz)/1
  sincos/1 -> Mux/1
  sincos/2 -> Mux/2
  Mux/1 -> Fcn11/1, Fcn12/1, Fcn13/1, Fcn21/1, Fcn32/1, Fcn33/1, Fcn31/1, Fcn23/1, Fcn22/1
  Fcn11/1 -> Create 3x3 Matrix/1
  Fcn12/1 -> Create 3x3 Matrix/2
  Fcn13/1 -> Create 3x3 Matrix/3
  Fcn31/1 -> Create 3x3 Matrix/7
  Fcn22/1 -> Create 3x3 Matrix/5
  Fcn32/1 -> Create 3x3 Matrix/8
  Fcn33/1 -> Create 3x3 Matrix/9
  Fcn21/1 -> Create 3x3 Matrix/4
  Fcn23/1 -> Create 3x3 Matrix/6

== system SM_Offshore_Windturbine/WIND TURBINE/ROTOR LOADS/Aerodynamic Loads/Blade 2/BEM/Node/Relative to absolute node/Subsystem ==
  Constant6 : Constant  Value=12
  Constant8 : Constant  Value=12.083
  Constant9 : Constant  Value=0.5
  Product3 : Product  Inputs=3
  X_iniz : Outport
  wires:
  Product3/1 -> X_iniz/1
  Constant8/1 -> Product3/2
  Constant6/1 -> Product3/3
  Constant9/1 -> Product3/1

== system SM_Offshore_Windturbine/WIND TURBINE/ROTOR LOADS/Aerodynamic Loads/Blade 3/BEM/Node/Relative to absolute node/3D rotation matirx ==
  "[rx; ry; rz]" : Inport  PortDimensions=3
  Create 3x3 Matrix : sharedutil/Create 3x3 Matrix  aMode=aMode
      settings: SourceProductBaseCode=AE,PW,DR,MT,UV,VE
  Fcn11 : Fcn  Expr=u(5)*u(6)
  Fcn12 : Fcn  Expr=u(6)*u(1)*u(2) - u(4)*u(3)
  Fcn13 : Fcn  Expr=u(4)*u(6)*u(2) + u(1)*u(3)
  Fcn21 : Fcn  Expr=u(5)*u(3)
  Fcn22 : Fcn  Expr=u(4)*u(6) + u(1)*u(2) *u(3)
  Fcn23 : Fcn  Expr=-u(6)*u(1) + u(4)*u(2) *u(3)
  Fcn31 : Fcn  Expr=-u(2)
  Fcn32 : Fcn  Expr=u(5)*u(1)
  Fcn33 : Fcn  Expr=u(4)*u(5)
  Mux : Mux  Inputs=2
  sincos : Trigonometry  Operator=sincos
  R(rx,ry,rz) : Outport  PortDimensions=[3,3]  VectorParamsAs1DForOutWhenUnconnected=off
  wires:
  "[rx; ry; rz]"/1 -> sincos/1
  Create 3x3 Matrix/1 -> R(rx,ry,rz)/1
  sincos/1 -> Mux/1
  sincos/2 -> Mux/2
  Mux/1 -> Fcn11/1, Fcn12/1, Fcn13/1, Fcn21/1, Fcn32/1, Fcn33/1, Fcn31/1, Fcn23/1, Fcn22/1
  Fcn11/1 -> Create 3x3 Matrix/1
  Fcn12/1 -> Create 3x3 Matrix/2
  Fcn13/1 -> Create 3x3 Matrix/3
  Fcn31/1 -> Create 3x3 Matrix/7
  Fcn22/1 -> Create 3x3 Matrix/5
  Fcn32/1 -> Create 3x3 Matrix/8
  Fcn33/1 -> Create 3x3 Matrix/9
  Fcn21/1 -> Create 3x3 Matrix/4
  Fcn23/1 -> Create 3x3 Matrix/6

== system SM_Offshore_Windturbine/WIND TURBINE/ROTOR LOADS/Aerodynamic Loads/Blade 3/BEM/Node/Relative to absolute node/Subsystem ==
  Constant6 : Constant  Value=12
  Constant8 : Constant  Value=12.083
  Constant9 : Constant  Value=0.5
  Product3 : Product  Inputs=3
  X_iniz : Outport
  wires:
  Product3/1 -> X_iniz/1
  Constant8/1 -> Product3/2
  Constant6/1 -> Product3/3
  Constant9/1 -> Product3/1

== matlab function SM_Offshore_Windturbine/WIND TURBINE/ROTOR LOADS/Aerodynamic Loads/Blade 1/Post_processing ==
  data: AIF input; AIF output; TIF input; TIF output
function [AIF,TIF] = Post_processing(AIF,TIF)
    for i=1:19
        if isnan(AIF(i))>0
            if i==19
                AIF(i)=AIF(i-1);
                TIF(i)=TIF(i-1);
            elseif i==1
                for j=i+1:19
                if isnan(AIF(j))==0
                AIF(i)=AIF(j);
                TIF(i)=TIF(j);
                break                
                end
                end
            else 
                for j=i+1:19
                if isnan(AIF(j))==0
                AIF(i)=AIF(i-1)+(AIF(j)-AIF(i-1))/(j-i);
                TIF(i)=TIF(i-1)+(TIF(j)-TIF(i-1))/(j-i);
                break 
                elseif j==19 && isnan(AIF(j))==1
                        AIF(i)=AIF(i-1);
                        TIF(i)=TIF(i-1);
                end
                end
            end
end
end          
end

== matlab function SM_Offshore_Windturbine/WIND TURBINE/ROTOR LOADS/Aerodynamic Loads/Blade 2/Post_processing ==
  data: AIF input; AIF output; TIF input; TIF output
function [AIF,TIF] = Post_processing(AIF,TIF)
    for i=1:19
        if isnan(AIF(i))>0
            if i==19
                AIF(i)=AIF(i-1);
                TIF(i)=TIF(i-1);
            elseif i==1
                for j=i+1:19
                if isnan(AIF(j))==0
                AIF(i)=AIF(j);
                TIF(i)=TIF(j);
                break                
                end
                end
            else 
                for j=i+1:19
                if isnan(AIF(j))==0
                AIF(i)=AIF(i-1)+(AIF(j)-AIF(i-1))/(j-i);
                TIF(i)=TIF(i-1)+(TIF(j)-TIF(i-1))/(j-i);
                break 
                elseif j==19 && isnan(AIF(j))==1
                        AIF(i)=AIF(i-1);
                        TIF(i)=TIF(i-1);
                end
                end
            end
end
end          
end

== matlab function SM_Offshore_Windturbine/WIND TURBINE/ROTOR LOADS/Aerodynamic Loads/Blade 3/Post_processing ==
  data: AIF input; AIF output; TIF input; TIF output
function [AIF,TIF] = Post_processing(AIF,TIF)
    for i=1:19
        if isnan(AIF(i))>0
            if i==19
                AIF(i)=AIF(i-1);
                TIF(i)=TIF(i-1);
            elseif i==1
                for j=i+1:19
                if isnan(AIF(j))==0
                AIF(i)=AIF(j);
                TIF(i)=TIF(j);
                break                
                end
                end
            else 
                for j=i+1:19
                if isnan(AIF(j))==0
                AIF(i)=AIF(i-1)+(AIF(j)-AIF(i-1))/(j-i);
                TIF(i)=TIF(i-1)+(TIF(j)-TIF(i-1))/(j-i);
                break 
                elseif j==19 && isnan(AIF(j))==1
                        AIF(i)=AIF(i-1);
                        TIF(i)=TIF(i-1);
                end
                end
            end
end
end          
end

== matlab function SM_Offshore_Windturbine/WIND TURBINE/ROTOR LOADS/Aerodynamic Loads/Integration ==
  data: Azimuth input; zNods input; RotTrq output; pN1 input; pT1 input; pN2 input; pT2 input; pN3 input; pT3 input; AeroLoads output
function [RotTrq,AeroLoads]  = Integration(Azimuth,zNods, pN1,pT1,pN2,pT2,pN3,pT3)

RotThr1 = trapz(zNods,pN1);
RotThr2 = trapz(zNods,pN2);
RotThr3 = trapz(zNods,pN3);
RotThr = RotThr1+RotThr2+RotThr3;

RotTrq1 = trapz(zNods,pT1.*zNods);
RotTrq2 = trapz(zNods,pT2.*zNods);
RotTrq3 = trapz(zNods,pT3.*zNods);
RotTrq = RotTrq1+RotTrq2+RotTrq3;

Ft1 = trapz(zNods,pT1);
Ft2 = trapz(zNods,pT2);
Ft3 = trapz(zNods,pT3);

FyAero = -(Ft1+Ft2*cos(120*pi/180)+Ft3*cos(240*pi/180));
FzAero = -(Ft2*sin(120*pi/180)+Ft3*sin(240*pi/180));

MzAero2 = trapz(zNods,pN2.*(zNods*sin(120*pi/180)));
MzAero3 = trapz(zNods,pN3.*(zNods*sin(240*pi/180)));
MzAero = MzAero2+MzAero3;

MyAero1 = trapz(zNods,pN1.*(zNods));
MyAero2 = trapz(zNods,pN2.*(zNods*cos(120*pi/180)));
MyAero3 = trapz(zNods,pN3.*(zNods*cos(240*pi/180)));
MyAero = MyAero1+MyAero2+MyAero3;

Fy=FyAero*cos(Azimuth)-FzAero*sin(Azimuth);
Fz=FyAero*sin(Azimuth)+FzAero*cos(Azimuth);
My=MyAero*cos(Azimuth)-MzAero*sin(Azimuth);
Mz=MyAero*sin(Azimuth)+MzAero*cos(Azimuth);

AeroLoads = [RotThr;Fy;Fz;RotTrq;My;Mz];
end
